simulink model "simulation_model_5"  (R2022a)
settings: Solver=ode3  StartTime=0.0  StopTime=Tsim  FixedStep=DTsim  RelTol=1e-3  EnableMultiTasking=on
values from neighbouring files (symbols this model uses):
  d1_step_final_value = 0.1*g    (= 0.981)    [simulation_script.m]
  d1_step_initial_value = 0    [simulation_script.m]
  d1_step_start = 5    [simulation_script.m]
  d1_step_stop = Tsim+1    (= 31)    [simulation_script.m]
  d2_step_final_value = g    (= 9.81)    [simulation_script.m]
  d2_step_initial_value = 0    [simulation_script.m]
  d2_step_start = 10    [simulation_script.m]
  d2_step_stop = Tsim+1    (= 31)    [simulation_script.m]
  DTsim = 0.01    [simulation_script.m]
  f = 0.1    [simulation_script.m]
  g = 9.81    [simulation_script.m]
  J = 0.2    [simulation_script.m]
  kd_gx = [2*xi*omega_]    [simulation_script.m]
  kd_gz = [2*xi*omega_]    [simulation_script.m]
  ki_x = [0.00001]    [simulation_script.m]
  ki_z = [0.00001]    [simulation_script.m]
  kp_gx = [omega_^2]    [simulation_script.m]
  kp_gz = [omega_^2]    [simulation_script.m]
  kp_vx = [3/Trep]    [simulation_script.m]
  kp_vz = [3/Trep]    [simulation_script.m]
  kp_x = [3/Trep]    [simulation_script.m]
  kp_z = [3/Trep]    [simulation_script.m]
  Lmax = 200    [simulation_script.m]
  Lmin = 0    [simulation_script.m]
  m = 10    [simulation_script.m]
  tau = 0.1    [simulation_script.m]
  Tmax = 0.035    [simulation_script.m]
  Tmin = -0.035    [simulation_script.m]
settings Model: Creator=mouyon  LastModifiedBy=leewh
settings SolverCC: AlgebraicLoopSolver=TrustRegion
settings DataIOCC: LimitDataPoints=on  SaveFormat=Array  SignalLoggingSaveFormat=ModelDataLogs  ReturnWorkspaceOutputs=off
settings OptimizationCC: DefaultParameterBehavior=Inlined  BufferReuse=off  ExpressionDepthLimit=2147483647  InitFltsAndDblsToZero=on  LifeSpan=inf
settings DebuggingCC: UnderspecifiedInitializationDetection=Classic  MergeDetectMultiDrivingBlocksExec=none  SolverPrmCheckMsg=warning  FcnCallInpInsideContextMsg=warning  UnconnectedInputMsg=warning  UnconnectedOutputMsg=warning  UnconnectedLineMsg=warning  AllowSymbolicDim=off  StateNameClashWarn=warning  InitInArrayFormatMsg=none  SFUnexpectedBacktrackingDiag=warning  SFNoUnconditionalDefaultTransitionDiag=warning  SFExecutionAtInitializationDiag=none  ArithmeticOperatorsInVariantConditions=warning
settings HardwareCC: ProdBitPerPointer=32  ProdBitPerSizeT=32  ProdBitPerPtrDiffT=32  ProdLargestAtomicFloat=None  ProdIntDivRoundTo=Undefined  ProdEndianess=Unspecified  ProdWordSize=32  ProdHWDeviceType=32-bit Generic
settings ModelReferenceCC: PropagateSignalLabelsOutOfModel=off
settings SFSimCC: SimUseLocalCustomCode=off  CustomCodeUndefinedFunction=UseInterfaceOnly
settings RTWCC: RTWUseLocalCustomCode=off
settings CodeAppCC: StateflowObjectComments=on
settings GRTTargetCC: TargetLangStandard=C89/C90 (ANSI)  CombineOutputUpdateFcns=off  GRTInterface=on
settings ConfigComp: CovMetricSettings=dw  CovSaveCumulativeToWorkspaceVar=on  CovSaveSingleToWorkspaceVar=on  CovExternalEMLEnable=off

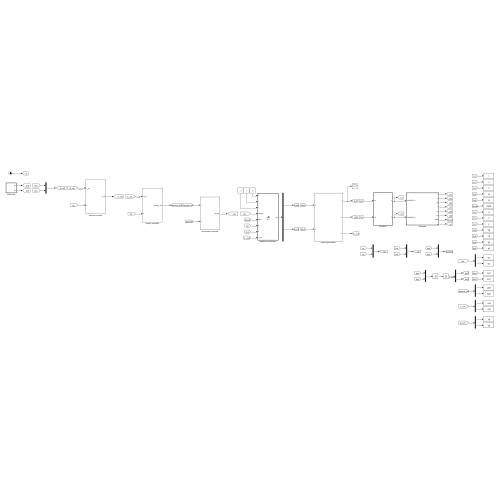
[thumbnail: Simulink's stored preview of the top-level diagram]
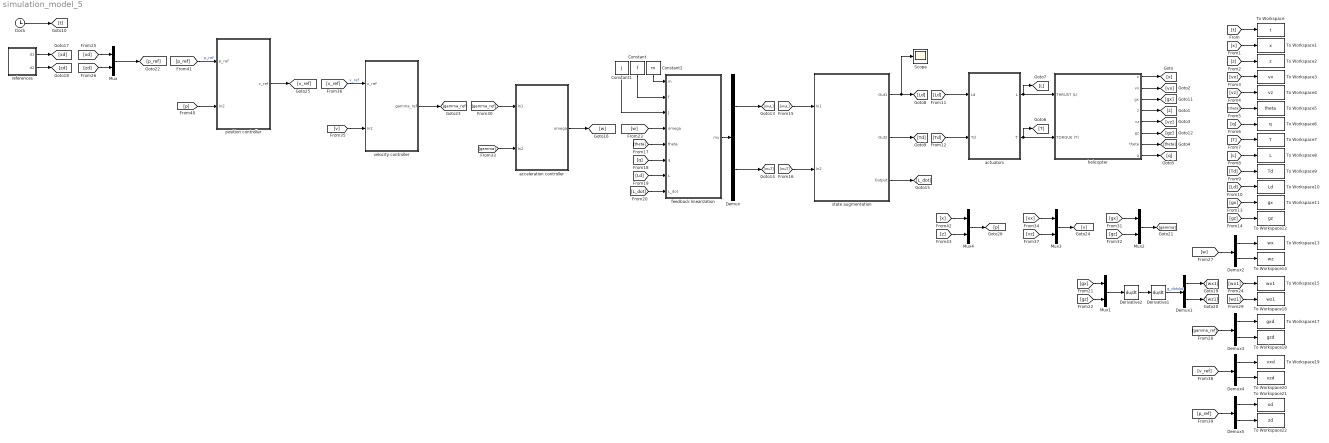
== system simulation_model_5 ==
  Clock : Clock
  Constant : Constant  Value=f
  Constant1 : Constant  Value=J
  Constant2 : Constant  Value=m
  Demux{,1..5} (6 alike) : Demux  Outputs=2
  Derivative1 : Derivative
  Derivative2 : Derivative
  Mux{,1..4} (5 alike) : Mux  Inputs=2
  Scope : Scope
  To Workspace : ToWorkspace  VariableName=t  SampleTime=-1
  To Workspace1 : ToWorkspace  VariableName=x  SampleTime=-1
  To Workspace10 : ToWorkspace  VariableName=Ld  SampleTime=-1
  To Workspace11 : ToWorkspace  VariableName=gx  SampleTime=-1
  To Workspace12 : ToWorkspace  VariableName=gz  SampleTime=-1
  To Workspace13 : ToWorkspace  VariableName=wx  SampleTime=-1
  To Workspace14 : ToWorkspace  VariableName=wz  SampleTime=-1
  To Workspace15 : ToWorkspace  VariableName=wx1  SampleTime=-1
  To Workspace16 : ToWorkspace  VariableName=wz1  SampleTime=-1
  To Workspace17 : ToWorkspace  VariableName=gxd  SampleTime=-1
  To Workspace18 : ToWorkspace  VariableName=gzd  SampleTime=-1
  To Workspace19 : ToWorkspace  VariableName=vxd  SampleTime=-1
  To Workspace2 : ToWorkspace  VariableName=z  SampleTime=-1
  To Workspace20 : ToWorkspace  VariableName=vzd  SampleTime=-1
  To Workspace21 : ToWorkspace  VariableName=xd  SampleTime=-1
  To Workspace22 : ToWorkspace  VariableName=zd  SampleTime=-1
  To Workspace3 : ToWorkspace  VariableName=vx  SampleTime=-1
  To Workspace4 : ToWorkspace  VariableName=vz  SampleTime=-1
  To Workspace5 : ToWorkspace  VariableName=theta  SampleTime=-1
  To Workspace6 : ToWorkspace  VariableName=q  SampleTime=-1
  To Workspace7 : ToWorkspace  VariableName=T  SampleTime=-1
  To Workspace8 : ToWorkspace  VariableName=L  SampleTime=-1
  To Workspace9 : ToWorkspace  VariableName=Td  SampleTime=-1
  acceleration controller : Subsystem
  actuators : Subsystem  TreatAsAtomicUnit=on
  feedback linearization : MATLAB Function  TreatAsAtomicUnit=on
  helicopter : Subsystem  TreatAsAtomicUnit=on
  position controller : Subsystem
  references : Subsystem  TreatAsAtomicUnit=on
  state augmentation : Subsystem
  velocity controller : Subsystem
  wires:
  helicopter/1(x) -> [x]
  helicopter/5(vz) -> [vz]
  helicopter/7(theta) -> [theta]
  helicopter/8(q) -> [q]
  Clock/1 -> [t]
  [t] -> To Workspace/1
  [x] -> To Workspace1/1
  [z] -> To Workspace2/1
  [vx] -> To Workspace3/1
  [vz] -> To Workspace4/1
  [theta] -> To Workspace5/1
  [q] -> To Workspace6/1
  [T] -> To Workspace7/1
  [L] -> To Workspace8/1
  [Td] -> To Workspace9/1
  [Ld] -> To Workspace10/1
  [Ld] -> actuators/1(Ld)
  [Td] -> actuators/2(Td)
  helicopter/2(vx) -> [vx]
  helicopter/4(z) -> [z]
  helicopter/3(gx) -> [gx]
  helicopter/6(gz) -> [gz]
  [gx] -> To Workspace11/1
  [gz] -> To Workspace12/1
  actuators/1(L) -> helicopter/1(THRUST (L)), [L]
  actuators/2(T) -> helicopter/2(TORQUE (T)), [T]
  [muL] -> state augmentation/1(In1)
  [muT] -> state augmentation/2(In2)
  state augmentation/1(Out1) -> Scope/1, [Ld]
  state augmentation/2(Out2) -> [Td]
  feedback linearization/1(mu) -> Demux/1
  Demux/1 -> [muL]
  Demux/2 -> [muT]
  Constant/1 -> feedback linearization/2(f)
  Constant1/1 -> feedback linearization/3(J)
  [theta] -> feedback linearization/5(theta)
  [q] -> feedback linearization/6(q)
  [Ld] -> feedback linearization/7(L)
  state augmentation/3(Output) -> [L_dot]
  [L_dot] -> feedback linearization/8(L_dot)
  Constant2/1 -> feedback linearization/1(m)
  [w] -> feedback linearization/4(omega)
  references/1(d1) -> [xd]
  references/2(d2) -> [zd]
  [xd] -> Mux/1
  [zd] -> Mux/2
  Demux2/1 -> To Workspace13/1
  Demux2/2 -> To Workspace14/1
  [gz] -> Mux1/2
  Derivative2/1 -> Derivative1/1
  Mux1/1 -> Derivative2/1
  [gx] -> Mux1/1
  Derivative1/1 -> Demux1/1  "g_dotdot"
  Demux1/1 -> [wx1]
  Demux1/2 -> [wz1]
  [wx1] -> To Workspace15/1
  [wz1] -> To Workspace16/1
  [gamma_ref] -> acceleration controller/1(In1)
  [gamma] -> acceleration controller/2(In2)
  Mux/1 -> [p_ref]
  acceleration controller/1(omega) -> [w]
  Mux2/1 -> [gamma]
  [gx] -> Mux2/1
  [gz] -> Mux2/2
  [w] -> Demux2/1
  Demux3/2 -> To Workspace18/1
  Demux3/1 -> To Workspace17/1
  velocity controller/1(gamma_ref) -> [gamma_ref]
  [v_ref] -> velocity controller/1(v_ref)  "v_ref"
  [v] -> velocity controller/2(In2)
  [gamma_ref] -> Demux3/1
  [vx] -> Mux3/1
  Mux3/1 -> [v]
  [vz] -> Mux3/2
  [p_ref] -> position controller/1(p_ref)  "p_ref"
  position controller/1(v_ref) -> [v_ref]
  [p] -> position controller/2(In2)
  [z] -> Mux4/2
  Mux4/1 -> [p]
  [x] -> Mux4/1
  [v_ref] -> Demux4/1
  Demux4/1 -> To Workspace19/1
  Demux4/2 -> To Workspace20/1
  Demux5/2 -> To Workspace22/1
  Demux5/1 -> To Workspace21/1
  [p_ref] -> Demux5/1

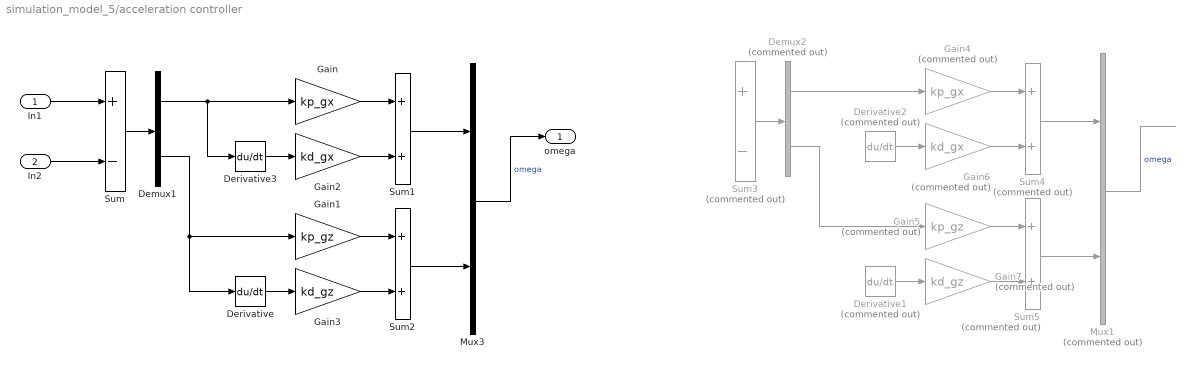
== system simulation_model_5/acceleration controller ==
  In1 : Inport
  In2 : Inport  Port=2
  Demux1 : Demux  Outputs=2
  Demux2 : Demux  Commented=on  Outputs=2
  Derivative : Derivative
  Derivative1 : Derivative  Commented=on
  Derivative2 : Derivative  Commented=on
  Derivative3 : Derivative
  Gain : Gain  Gain=kp_gx
  Gain1 : Gain  Gain=kp_gz
  Gain2 : Gain  Gain=kd_gx
  Gain3 : Gain  Gain=kd_gz
  Gain4 : Gain  Commented=on  Gain=kp_gx
  Gain5 : Gain  Commented=on  Gain=kp_gz
  Gain6 : Gain  Commented=on  Gain=kd_gx
  Gain7 : Gain  Commented=on  Gain=kd_gz
  Mux1 : Mux  Commented=on  Inputs=2
  Mux3 : Mux  Inputs=2
  Sum : Sum  Inputs=+-
  Sum1 : Sum
  Sum2 : Sum
  Sum3 : Sum  Commented=on  Inputs=+-
  Sum4 : Sum  Commented=on
  Sum5 : Sum  Commented=on
  omega : Outport
  wires:
  Gain2/1 -> Sum1/2
  Derivative/1 -> Gain3/1
  Sum1/1 -> Mux3/1
  Demux1/1 -> Gain/1, Derivative3/1
  Gain1/1 -> Sum2/1
  Sum2/1 -> Mux3/2
  Gain/1 -> Sum1/1
  In1/1 -> Sum/1
  Derivative3/1 -> Gain2/1
  Demux1/2 -> Derivative/1, Gain1/1
  Gain3/1 -> Sum2/2
  Sum/1 -> Demux1/1
  Mux3/1 -> omega/1  "omega"
  In2/1 -> Sum/2
  Mux1/1 -> ?  "omega"
  Derivative2/1 -> Gain6/1
  ? -> Derivative1/1, Derivative2/1, Sum3/2
  ? -> Sum3/1
  Gain7/1 -> Sum5/2
  Demux2/2 -> Gain5/1
  Sum3/1 -> Demux2/1
  Derivative1/1 -> Gain7/1
  Gain5/1 -> Sum5/1
  Sum5/1 -> Mux1/2
  Gain4/1 -> Sum4/1
  Gain6/1 -> Sum4/2
  Demux2/1 -> Gain4/1
  Sum4/1 -> Mux1/1

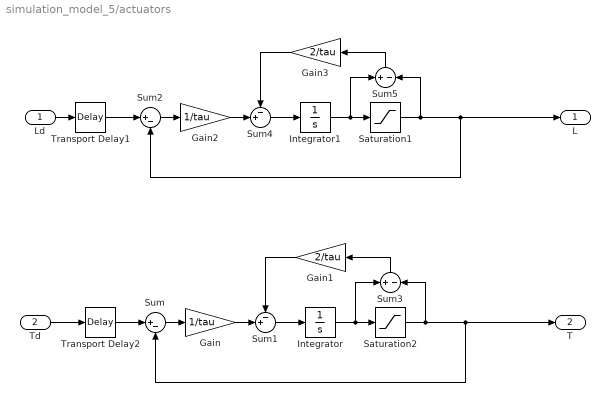
== system simulation_model_5/actuators ==
  Ld : Inport
  Td : Inport  Port=2
  Gain : Gain  Gain=1/tau
  Gain1 : Gain  Gain=2/tau
  Gain2 : Gain  Gain=1/tau
  Gain3 : Gain  Gain=2/tau
  Integrator : Integrator
  Integrator1 : Integrator  InitialCondition=m*g
  Saturation1 : Saturate  UpperLimit=Lmax  LowerLimit=Lmin
  Saturation2 : Saturate  UpperLimit=Tmax  LowerLimit=Tmin
  Sum : Sum  Inputs=|+-
  Sum1 : Sum  Inputs=-+|
  Sum2 : Sum  Inputs=|+-
  Sum3 : Sum  Inputs=+|-  SaturateOnIntegerOverflow=on
  Sum4 : Sum  Inputs=-+|
  Sum5 : Sum  Inputs=+|-  SaturateOnIntegerOverflow=on
  Transport Delay1 : TransportDelay  DelayTime=DTsim  InitialOutput=m*g
  Transport Delay2 : TransportDelay  DelayTime=DTsim
  L : Outport
  T : Outport  Port=2
  wires:
  Integrator/1 -> Sum3/1, Saturation2/1
  Sum/1 -> Gain/1
  Td/1 -> Transport Delay2/1
  Sum3/1 -> Gain1/1
  Gain/1 -> Sum1/2
  Sum1/1 -> Integrator/1
  Integrator1/1 -> Saturation1/1, Sum5/1
  Sum2/1 -> Gain2/1
  Ld/1 -> Transport Delay1/1
  Saturation1/1 -> Sum2/2, L/1, Sum5/2
  Sum5/1 -> Gain3/1
  Gain2/1 -> Sum4/2
  Sum4/1 -> Integrator1/1
  Gain3/1 -> Sum4/1
  Gain1/1 -> Sum1/1
  Saturation2/1 -> Sum/2, T/1, Sum3/2
  Transport Delay1/1 -> Sum2/1
  Transport Delay2/1 -> Sum/1

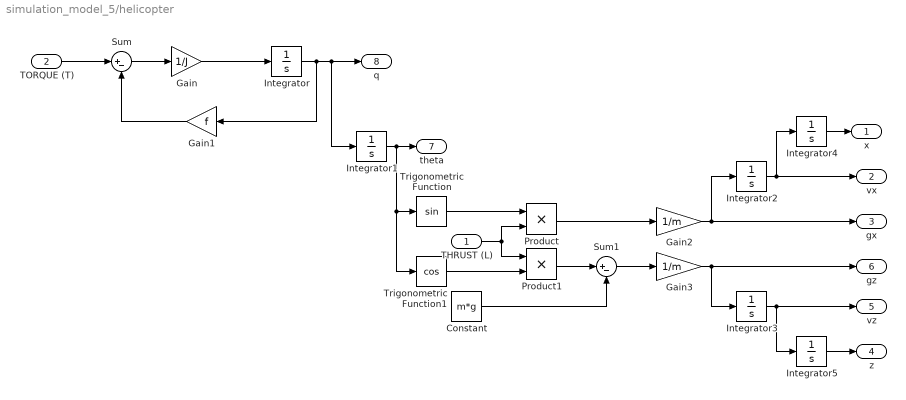
== system simulation_model_5/helicopter ==
  THRUST (L) : Inport
  TORQUE (T) : Inport  Port=2
  Constant : Constant  Value=m*g
  Gain : Gain  Gain=1/J
  Gain1 : Gain  Gain=f
  Gain2 : Gain  Gain=1/m
  Gain3 : Gain  Gain=1/m
  Integrator{,1..5} (6 alike) : Integrator
  Product : Product  RndMeth=Zero
  Product1 : Product  RndMeth=Zero
  Sum : Sum  Inputs=|+-
  Sum1 : Sum  Inputs=|+-
  Trigonometric Function : Trigonometry
  Trigonometric Function1 : Trigonometry  Operator=cos
  x : Outport
  vx : Outport  Port=2
  gx : Outport  Port=3
  z : Outport  Port=4
  vz : Outport  Port=5
  gz : Outport  Port=6
  theta : Outport  Port=7
  q : Outport  Port=8
  wires:
  Integrator/1 -> Gain1/1, q/1, Integrator1/1
  Gain/1 -> Integrator/1
  Gain1/1 -> Sum/2
  Sum/1 -> Gain/1
  TORQUE (T)/1 -> Sum/1
  Integrator1/1 -> theta/1, Trigonometric Function/1, Trigonometric Function1/1
  Trigonometric Function/1 -> Product/1
  THRUST (L)/1 -> Product/2, Product1/1
  Trigonometric Function1/1 -> Product1/2
  Product/1 -> Gain2/1
  Product1/1 -> Sum1/1
  Constant/1 -> Sum1/2
  Gain3/1 -> gz/1, Integrator3/1
  Sum1/1 -> Gain3/1
  Integrator2/1 -> vx/1, Integrator4/1
  Integrator3/1 -> vz/1, Integrator5/1
  Integrator4/1 -> x/1
  Integrator5/1 -> z/1
  Gain2/1 -> gx/1, Integrator2/1

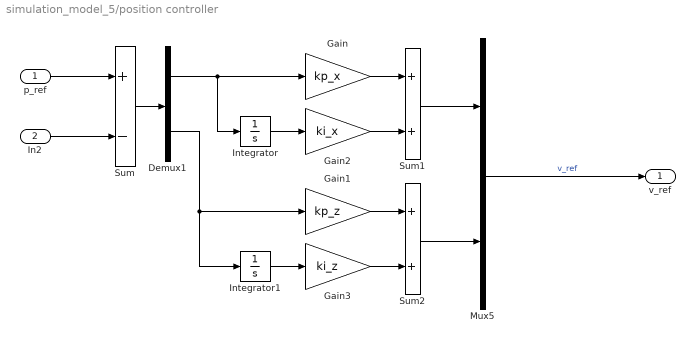
== system simulation_model_5/position controller ==
  p_ref : Inport
  In2 : Inport  Port=2
  Demux1 : Demux  Outputs=2
  Gain : Gain  Gain=kp_x
  Gain1 : Gain  Gain=kp_z
  Gain2 : Gain  Gain=ki_x
  Gain3 : Gain  Gain=ki_z
  Integrator : Integrator
  Integrator1 : Integrator
  Mux5 : Mux  Inputs=2
  Sum : Sum  Inputs=+-
  Sum1 : Sum
  Sum2 : Sum
  v_ref : Outport
  wires:
  Gain2/1 -> Sum1/2
  Demux1/1 -> Integrator/1, Gain/1
  Sum2/1 -> Mux5/2
  Sum1/1 -> Mux5/1
  In2/1 -> Sum/2
  Demux1/2 -> Integrator1/1, Gain1/1
  Integrator1/1 -> Gain3/1
  Integrator/1 -> Gain2/1
  p_ref/1 -> Sum/1
  Gain/1 -> Sum1/1
  Sum/1 -> Demux1/1
  Gain1/1 -> Sum2/1
  Gain3/1 -> Sum2/2
  Mux5/1 -> v_ref/1  "v_ref"

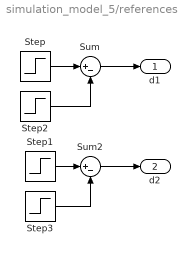
== system simulation_model_5/references ==
  Step : Step  Time=d1_step_start  Before=d1_step_initial_value  After=d1_step_final_value  SampleTime=0
  Step1 : Step  Time=d2_step_start  Before=d2_step_initial_value  After=d2_step_final_value  SampleTime=0
  Step2 : Step  Time=d1_step_stop  After=d1_step_final_value  SampleTime=0
  Step3 : Step  Time=d2_step_stop  After=d2_step_final_value  SampleTime=0
  Sum : Sum  Inputs=|+-
  Sum2 : Sum  Inputs=|+-
  d1 : Outport
  d2 : Outport  Port=2
  wires:
  Step/1 -> Sum/1
  Step2/1 -> Sum/2
  Step1/1 -> Sum2/1
  Sum/1 -> d1/1
  Sum2/1 -> d2/1
  Step3/1 -> Sum2/2

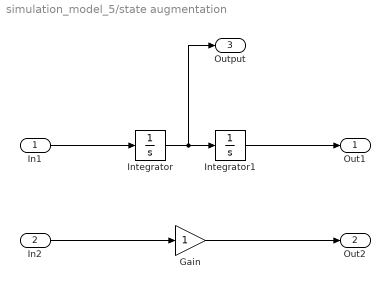
== system simulation_model_5/state augmentation ==
  In1 : Inport
  In2 : Inport  Port=2
  Gain : Gain
  Integrator : Integrator
  Integrator1 : Integrator  InitialCondition=m*g
  Out1 : Outport
  Out2 : Outport  Port=2
  Output : Outport  Port=3
  wires:
  Integrator/1 -> Output/1, Integrator1/1
  In1/1 -> Integrator/1
  In2/1 -> Gain/1
  Integrator1/1 -> Out1/1
  Gain/1 -> Out2/1

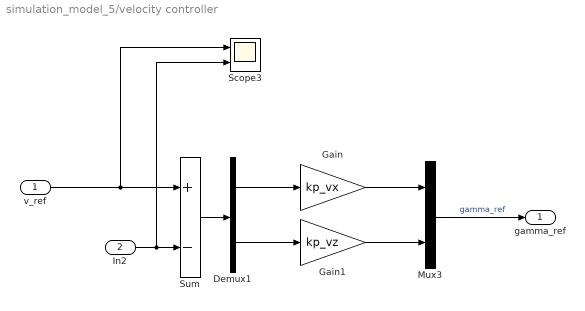
== system simulation_model_5/velocity controller ==
  v_ref : Inport
  In2 : Inport  Port=2
  Demux1 : Demux  Outputs=2
  Gain : Gain  Gain=kp_vx
  Gain1 : Gain  Gain=kp_vz
  Mux3 : Mux  Inputs=2
  Scope3 : Scope  NumInputPorts=2
  Sum : Sum  Inputs=+-
  gamma_ref : Outport
  wires:
  Gain/1 -> Mux3/1
  Mux3/1 -> gamma_ref/1  "gamma_ref"
  Gain1/1 -> Mux3/2
  Demux1/2 -> Gain1/1
  v_ref/1 -> Scope3/1, Sum/1
  In2/1 -> Scope3/2, Sum/2
  Sum/1 -> Demux1/1
  Demux1/1 -> Gain/1

== matlab function simulation_model_5/feedback linearization ==
  data: m input; f input; J input; omega input; theta input; q input; mu output; L input; L_dot input
function mu = fcn(m, f, J, omega, theta, q, L, L_dot)

% delta_inv_delta_zero  = [L*f*q/J*sin(2*theta) - L*q^2
%                     q*f*cos(2*theta) + 2*L_dot*J*q/L];

delta_inv_delta_zero  = [-L*q^2*cos(2*theta)
                         q*(2*J*L_dot/L - f + J*q*sin(2*theta))];

delta_inv = m*[      sin(theta),         cos(theta)
               (J/L)*cos(theta),  -(J/L)*sin(theta)]; 

mu = -delta_inv_delta_zero + delta_inv*omega;
